simulink model "Mod4VidAincomplete"  (R2022b)
settings: Solver=FixedStepAuto  StartTime=0.0  StopTime=inf  RelTol=1e-3  EnableMultiTasking=on
libraries: vexarmcortexlib x21, RoboticsPlayground x1, vexcommonlib x1
settings Model: Creator=carol  LastModifiedBy=carol
settings DataIOCC: LimitDataPoints=on  SignalLoggingSaveFormat=ModelDataLogs  ReturnWorkspaceOutputs=off
settings OptimizationCC: ExpressionDepthLimit=2147483647  LifeSpan=Inf  MaxStackSize=64  EfficientTunableParamExpr=on
settings DebuggingCC: UnderspecifiedInitializationDetection=Classic  MergeDetectMultiDrivingBlocksExec=none  InheritedTsInSrcMsg=none  FcnCallInpInsideContextMsg=warning  StateNameClashWarn=warning  SFUnexpectedBacktrackingDiag=warning  SFNoUnconditionalDefaultTransitionDiag=warning  SFExecutionAtInitializationDiag=none  SFMachineParentedDataDiag=warning  ArithmeticOperatorsInVariantConditions=warning
settings HardwareCC: ProdBitPerPointer=32  ProdBitPerSizeT=32  ProdBitPerPtrDiffT=32  ProdLargestAtomicInteger=Long  ProdLargestAtomicFloat=Double  ProdIntDivRoundTo=Undefined  ProdWordSize=32  ProdHWDeviceType=ARM Compatible->ARM Cortex
settings ModelReferenceCC: EnableRefExpFcnMdlSchedulingChecks=on  PropagateSignalLabelsOutOfModel=off
settings SFSimCC: MATLABDynamicMemAlloc=off  CustomCodeUndefinedFunction=UseInterfaceOnly
settings RTWCC: Description=Embedded Coder  SystemTargetFile=ert.tlc  HardwareBoard=ARM Cortex-based VEX Microcontroller  TemplateMakefile=ert_default_tmf  Toolchain=GNU Tools for VEX ARM Cortex
settings CodeAppCC: IgnoreCustomStorageClasses=off  CustomSymbolStrType=$N$R$M  StateflowObjectComments=on  InternalIdentifier=Classic
settings ERTTargetCC: CodeReplacementLibrary=GCC ARM Cortex-M3  MultiwordLength=2048  ConvertIfToSwitch=off  SuppressUnreachableDefaultCases=off

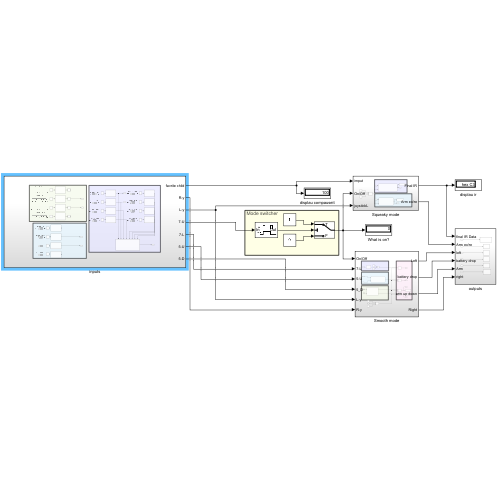
[thumbnail: Simulink's stored preview of the top-level diagram]
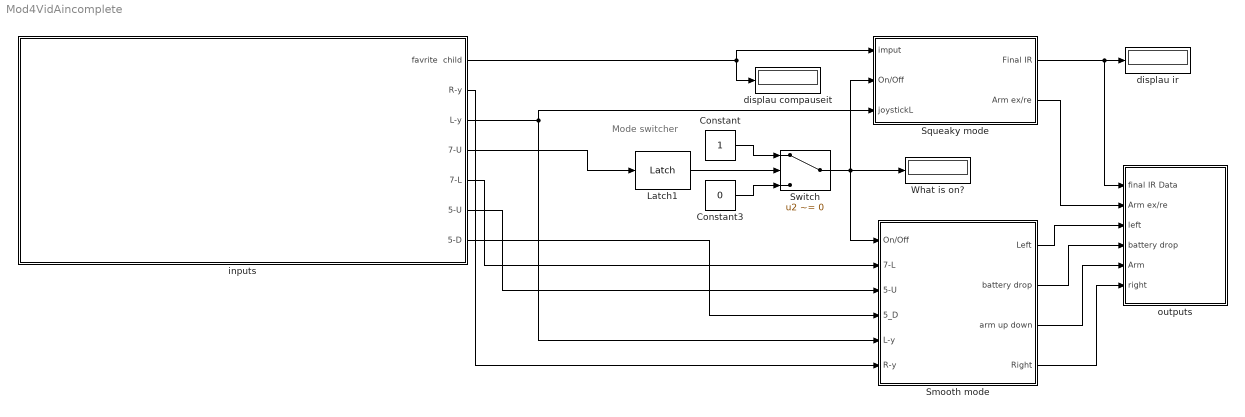
== system Mod4VidAincomplete ==
  note: Mode switcher
  Constant : Constant
  Constant3 : Constant  Value=0
  Latch1 : RoboticsPlayground/Utilities and Hardware/Latch  SystemSampleTime=-1  VariantActivationTime=update diagram  Latency=0  AutoFrameSizeCalculation=off
      settings: SourceProductName=Robotics Playground
  Smooth mode : Subsystem
  Squeaky mode : Subsystem
  Switch : Switch  Criteria=u2 ~= 0  SaturateOnIntegerOverflow=off  InputSameDT=off
  What is on? : Display
  displau compauseit : Display
  displau ir : Display
      settings: Format=hex (Stored Integer)
  inputs : Subsystem
  outputs : Subsystem
  wires:
  Switch/1 -> Squeaky mode/2(On/Off), What is on?/1, Smooth mode/1(On/Off)
  Constant3/1 -> Switch/3
  Latch1/1 -> Switch/2
  inputs/1(favrite  child) -> Squeaky mode/1(imput), displau compauseit/1
  inputs/4(7-U) -> Latch1/1
  Constant/1 -> Switch/1
  inputs/3(L-y) -> Squeaky mode/3(joystickL), Smooth mode/5(L-y)
  Smooth mode/1(Left) -> outputs/3(left)
  Smooth mode/2(battery drop) -> outputs/4(battery drop)
  Smooth mode/4(Right) -> outputs/6(right)
  Smooth mode/3(arm up down) -> outputs/5("Arm ")
  inputs/2(R-y) -> Smooth mode/6(R-y)
  inputs/7(5-D) -> Smooth mode/4(5_D)
  inputs/6(5-U) -> Smooth mode/3(5-U)
  inputs/5(7-L) -> Smooth mode/2(7-L)
  Squeaky mode/1(Final IR) -> displau ir/1, outputs/1(final IR Data)
  Squeaky mode/2(Arm ex/re) -> outputs/2(Arm ex/re)

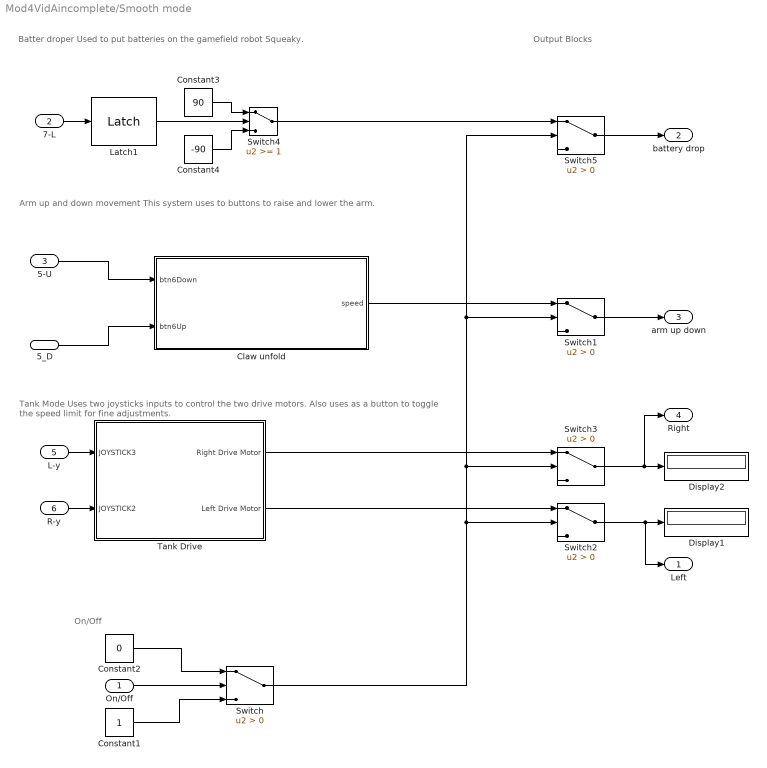
== system Mod4VidAincomplete/Smooth mode ==
  note: Output Blocks
  note: Batter droper
      | Used to put batteries on the gamefield robot Squeaky.
  note: Tank Mode
      | Uses two joysticks inputs to control the two drive motors. Also uses as a button
      | to toggle the speed limit for fine adjustments.
  note: Arm up and down movement
      | This system uses to buttons to raise and lower the arm.
  note: On/Off
  On/Off : Inport
  7-L : Inport  Port=2
  5-U : Inport  Port=3
  5_D : Inport  Port=4
  L-y : Inport  Port=5
  R-y : Inport  Port=6
  Claw unfold : Stateflow chart  TreatAsAtomicUnit=on
  Constant1 : Constant
  Constant2 : Constant  Value=0
  Constant3 : Constant  Value=90
  Constant4 : Constant  Value=-90
  Display1 : Display
  Display2 : Display
  Latch1 : vexcommonlib/Latch  output0=off  BlockPlatform=vexarmcortex
  Switch{,1..3,5} (5 alike) : Switch  Criteria=u2 > Threshold  SaturateOnIntegerOverflow=off  InputSameDT=off
  Switch4 : Switch  Threshold=1  SaturateOnIntegerOverflow=off  InputSameDT=off
  "Tank Drive " : Subsystem  TreatAsAtomicUnit=on
  Left : Outport
  battery drop : Outport  Port=2
  arm up down : Outport  Port=3
  Right : Outport  Port=4
  wires:
  Constant2/1 -> Switch/1
  On/Off/1 -> Switch/2
  5_D/1 -> Claw unfold/2(btn6Up)
  5-U/1 -> Claw unfold/1(btn6Down)
  Latch1/1 -> Switch4/2
  Constant4/1 -> Switch4/3
  R-y/1 -> "Tank Drive "/2(JOYSTICK2)
  "Tank Drive "/1(Right Drive Motor) -> Switch3/1
  L-y/1 -> "Tank Drive "/1(JOYSTICK3)
  7-L/1 -> Latch1/1
  Claw unfold/1(speed) -> Switch1/1
  Constant3/1 -> Switch4/1
  "Tank Drive "/2(Left Drive Motor) -> Switch2/1
  Switch4/1 -> Switch5/1
  Switch/1 -> Switch2/2, Switch3/2, Switch5/2, Switch1/2
  Switch5/1 -> battery drop/1
  Switch1/1 -> arm up down/1
  Switch3/1 -> Right/1, Display2/1
  Switch2/1 -> Left/1, Display1/1
  Constant1/1 -> Switch/3

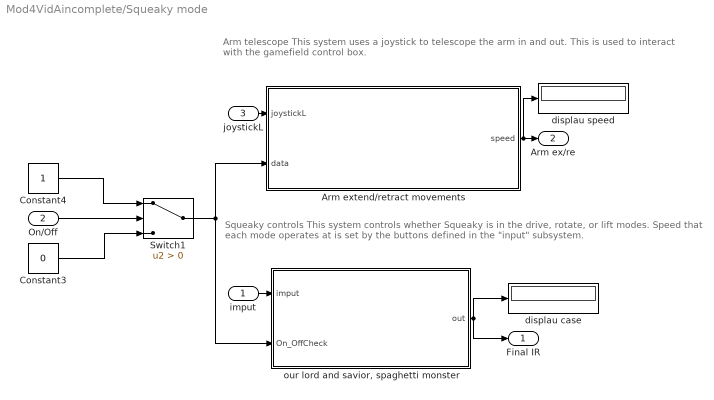
== system Mod4VidAincomplete/Squeaky mode ==
  note: Squeaky controls
      | This system controls whether Squeaky is in the drive, rotate, or lift modes.
      | Speed that each mode operates at is set by the buttons defined in the "input" subsystem.
  note: Arm telescope
      | This system uses a joystick to telescope the arm in and out.
      | This is used to interact with the gamefield control box.
  imput : Inport
  On/Off : Inport  Port=2
  joystickL : Inport  Port=3
  Arm extend/retract movements : Stateflow chart  TreatAsAtomicUnit=on
  Constant3 : Constant  Value=0
  Constant4 : Constant
  Switch1 : Switch  Criteria=u2 > Threshold  SaturateOnIntegerOverflow=off  InputSameDT=off
  displau case : Display
  displau speed : Display
  "our lord and savior, spaghetti monster" : Stateflow chart  TreatAsAtomicUnit=on
  Final IR : Outport
  Arm ex/re : Outport  Port=2
  wires:
  Switch1/1 -> Arm extend/retract movements/2(data), "our lord and savior, spaghetti monster"/2(On_OffCheck)
  imput/1 -> "our lord and savior, spaghetti monster"/1(imput)
  Constant3/1 -> Switch1/3
  joystickL/1 -> Arm extend/retract movements/1(joystickL)
  Arm extend/retract movements/1(speed) -> Arm ex/re/1, displau speed/1
  On/Off/1 -> Switch1/2
  Constant4/1 -> Switch1/1
  "our lord and savior, spaghetti monster"/1(out) -> Final IR/1, displau case/1

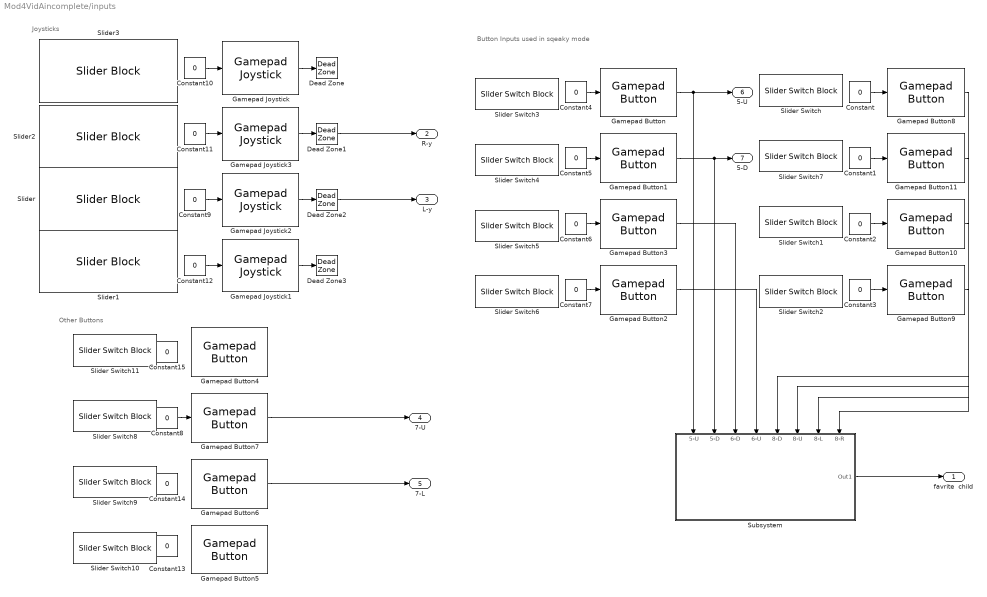
== system Mod4VidAincomplete/inputs ==
  note: Other Buttons
  note: Button Inputs used in sqeaky mode
  note: Joysticks
  Constant{,1..15} (16 alike) : Constant  Value=0
  Dead Zone{,1..3} (4 alike) : DeadZone  LowerValue=-10  UpperValue=10
  Gamepad Button : vexarmcortexlib/Gamepad/Gamepad Button  joystick=1  chan=5  button56=Up  button78=Down  SimulationIn=on  SampleTime=0.02
  Gamepad Button1 : vexarmcortexlib/Gamepad/Gamepad Button  joystick=1  chan=5  button56=Down  button78=Down  SimulationIn=on  SampleTime=0.02
  Gamepad Button10 : vexarmcortexlib/Gamepad/Gamepad Button  joystick=1  chan=8  button56=Up  button78=Left  SimulationIn=on  SampleTime=0.02
  Gamepad Button11 : vexarmcortexlib/Gamepad/Gamepad Button  joystick=1  chan=8  button56=Up  button78=Up  SimulationIn=on  SampleTime=0.02
  Gamepad Button2 : vexarmcortexlib/Gamepad/Gamepad Button  joystick=1  chan=6  button56=Up  button78=Down  SimulationIn=on  SampleTime=0.02
  Gamepad Button3 : vexarmcortexlib/Gamepad/Gamepad Button  joystick=1  chan=6  button56=Down  button78=Down  SimulationIn=on  SampleTime=0.02
  Gamepad Button4 : vexarmcortexlib/Gamepad/Gamepad Button  joystick=1  chan=7  button56=Up  button78=Down  SimulationIn=off  SampleTime=0.02
  Gamepad Button5 : vexarmcortexlib/Gamepad/Gamepad Button  joystick=1  chan=7  button56=Up  button78=Right  SimulationIn=off  SampleTime=0.02
  Gamepad Button6 : vexarmcortexlib/Gamepad/Gamepad Button  joystick=1  chan=7  button56=Up  button78=Left  SimulationIn=off  SampleTime=0.02
  Gamepad Button7 : vexarmcortexlib/Gamepad/Gamepad Button  joystick=1  chan=7  button56=Up  button78=Up  SimulationIn=on  SampleTime=0.02
  Gamepad Button8 : vexarmcortexlib/Gamepad/Gamepad Button  joystick=1  chan=8  button56=Up  button78=Down  SimulationIn=on  SampleTime=0.02
  Gamepad Button9 : vexarmcortexlib/Gamepad/Gamepad Button  joystick=1  chan=8  button56=Up  button78=Right  SimulationIn=on  SampleTime=0.02
  Gamepad Joystick : vexarmcortexlib/Gamepad/Gamepad Joystick  joystick=1  chan=1  SimulationIn=on  SampleTime=0.02
  Gamepad Joystick1 : vexarmcortexlib/Gamepad/Gamepad Joystick  joystick=1  chan=4  SimulationIn=on  SampleTime=0.02
  Gamepad Joystick2 : vexarmcortexlib/Gamepad/Gamepad Joystick  joystick=1  chan=3  SimulationIn=on  SampleTime=0.02
  Gamepad Joystick3 : vexarmcortexlib/Gamepad/Gamepad Joystick  joystick=1  chan=2  SimulationIn=on  SampleTime=0.02
  Slider{,1..3} (4 alike) : SliderBlock  ScaleMin=-180  ScaleMax=180
  Slider Switch{,1..11} (12 alike) : SliderSwitchBlock
      settings: Values={{'Off', 'On'}, [0 1]}
  Subsystem : Subsystem
      settings: PortSchema="{\"entries\":[{\"content\":{\"sides\":[{\"content\":{\"connectorIds\":[]},\"type\":\"ConnectorPlacement.EquallySpacedRectSide\",\"uuid\":\"9d2b5337-c4d4-4923-a699-a47fc21a7185\"},{\"content\":{\"connectorIds\":[\"Out1\"],\"side\":\"RIGHT\"},\"type\":\"ConnectorPlacement.EquallySpacedRectSide\",\"uuid\":\"56c06069-3940-4c56-b8fd-a4c3d4ffc63d\"},{\"content\":{\"connectorIds\":[\"In1\",\"In2\",\"In3\",\"In4\",\"In5\",\"In6\",\"In7\",\"In8\"],\"side\":\"TOP\"},\"type\":\"ConnectorPlacement.EquallySpacedRectSide\",\"uuid\":\"14368183-39e9-4405-bfbf-e8557249760c\"}]},\"type\":\"ConnectorPlacement.EquallySpacedConnector\",\"uuid\":\"5d0b0675-df6a-4749-851b-50901843da5f\"}],\"packageUris\":[\"http://schema.mathworks.com/mf0/Connector/R2020b\"],\"version\":\"1.0\"}"
  favrite  child : Outport
  R-y : Outport  Port=2
  L-y : Outport  Port=3
  7-U : Outport  Port=4
  7-L : Outport  Port=5
  5-U : Outport  Port=6
  5-D : Outport  Port=7
  wires:
  Gamepad Joystick/1 -> Dead Zone/1
  Gamepad Button7/1 -> 7-U/1
  Gamepad Button6/1 -> 7-L/1
  Constant/1 -> Gamepad Button8/1
  Constant1/1 -> Gamepad Button11/1
  Constant2/1 -> Gamepad Button10/1
  Constant3/1 -> Gamepad Button9/1
  Constant4/1 -> Gamepad Button/1
  Constant5/1 -> Gamepad Button1/1
  Constant7/1 -> Gamepad Button2/1
  Constant6/1 -> Gamepad Button3/1
  Constant8/1 -> Gamepad Button7/1
  Subsystem/1(Out1) -> favrite  child/1
  Constant9/1 -> Gamepad Joystick2/1
  Gamepad Button/1 -> 5-U/1, Subsystem/1(5-U)
  Gamepad Button1/1 -> 5-D/1, Subsystem/2(5-D)
  Gamepad Button3/1 -> Subsystem/3(6-D)
  Gamepad Button2/1 -> Subsystem/4(6-U)
  Gamepad Button8/1 -> Subsystem/5(8-D)
  Gamepad Button11/1 -> Subsystem/6(8-U)
  Gamepad Button10/1 -> Subsystem/7(8-L)
  Gamepad Button9/1 -> Subsystem/8(8-R)
  Constant12/1 -> Gamepad Joystick1/1
  Constant11/1 -> Gamepad Joystick3/1
  Constant10/1 -> Gamepad Joystick/1
  Gamepad Joystick3/1 -> Dead Zone1/1
  Gamepad Joystick2/1 -> Dead Zone2/1
  Dead Zone2/1 -> L-y/1
  Dead Zone1/1 -> R-y/1
  Gamepad Joystick1/1 -> Dead Zone3/1

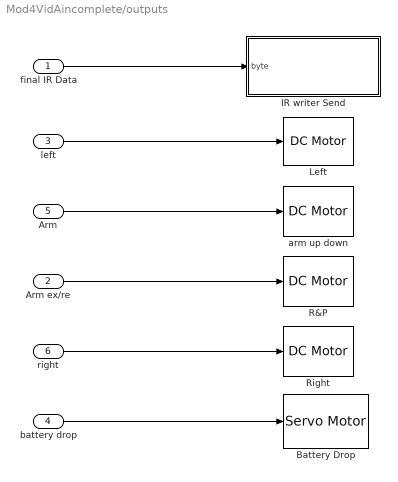
== system Mod4VidAincomplete/outputs ==
  final IR Data : Inport
  Arm ex/re : Inport  Port=2
  left : Inport  Port=3
  battery drop : Inport  Port=4
  "Arm " : Inport  Port=5
  right : Inport  Port=6
  Battery Drop : vexarmcortexlib/Actuators/Servo Motor  motor=3  scaleFactor=60/127  SimulationOut=off
  IR writer Send : Subsystem
  Left : vexarmcortexlib/Actuators/DC Motor  motor=2  scaleFactor=1/13.5  SimulationOut=off
  R&P : vexarmcortexlib/Actuators/DC Motor  motor=6  scaleFactor=1/13.5  SimulationOut=off
  Right : vexarmcortexlib/Actuators/DC Motor  motor=9  scaleFactor=1/13.5  SimulationOut=off
  arm up down : vexarmcortexlib/Actuators/DC Motor  motor=4  scaleFactor=1/13.5  SimulationOut=off
  wires:
  final IR Data/1 -> IR writer Send/1(byte)
  Arm ex/re/1 -> R&P/1
  left/1 -> Left/1
  battery drop/1 -> Battery Drop/1
  right/1 -> Right/1
  "Arm "/1 -> arm up down/1

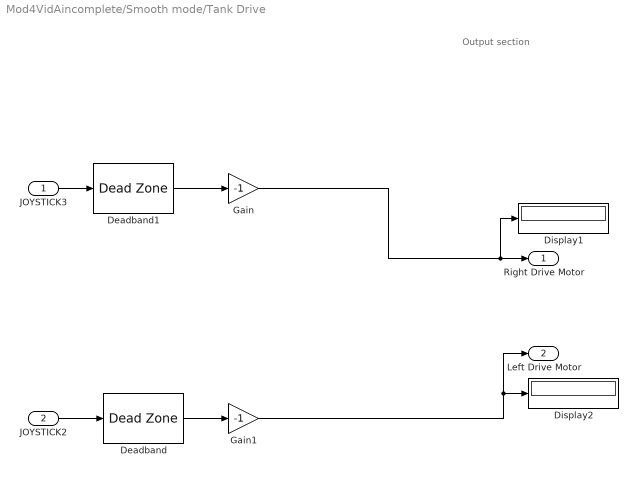
== system Mod4VidAincomplete/Smooth mode/Tank Drive  ==
  note: Output section
  JOYSTICK3 : Inport
  JOYSTICK2 : Inport  Port=2
  Deadband : DeadZone  LowerValue=-9  UpperValue=9
  Deadband1 : DeadZone  LowerValue=-9  UpperValue=9
  Display1 : Display
  Display2 : Display
  Gain : Gain  Gain=-1
  Gain1 : Gain  Gain=-1
  Right Drive Motor : Outport
  Left Drive Motor : Outport  Port=2
  wires:
  JOYSTICK3/1 -> Deadband1/1
  Gain/1 -> Display1/1, Right Drive Motor/1
  Gain1/1 -> Display2/1, Left Drive Motor/1
  JOYSTICK2/1 -> Deadband/1
  Deadband1/1 -> Gain/1
  Deadband/1 -> Gain1/1

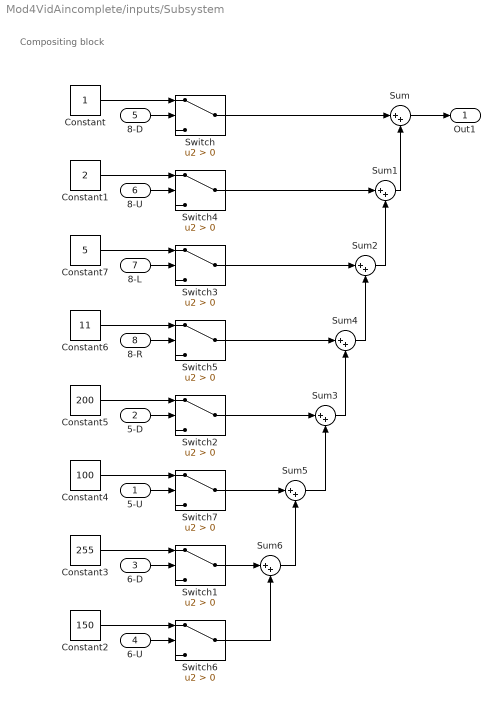
== system Mod4VidAincomplete/inputs/Subsystem ==
  note: Compositing block
  5-U : Inport
  5-D : Inport  Port=2
  6-D : Inport  Port=3
  6-U : Inport  Port=4
  8-D : Inport  Port=5
  8-U : Inport  Port=6
  8-L : Inport  Port=7
  8-R : Inport  Port=8
  Constant : Constant
  Constant1 : Constant  Value=2
  Constant2 : Constant  Value=150
  Constant3 : Constant  Value=255
  Constant4 : Constant  Value=100
  Constant5 : Constant  Value=200
  Constant6 : Constant  Value=11
  Constant7 : Constant  Value=5
  Sum{,1..6} (7 alike) : Sum  Inputs=|++
  Switch{,1..7} (8 alike) : Switch  Criteria=u2 > Threshold  SaturateOnIntegerOverflow=off  InputSameDT=off
  Out1 : Outport
  wires:
  8-D/1 -> Switch/2
  Sum/1 -> Out1/1
  Switch4/1 -> Sum1/1
  Sum1/1 -> Sum/2
  Switch3/1 -> Sum2/1
  Sum2/1 -> Sum1/2
  Switch5/1 -> Sum4/1
  Switch6/1 -> Sum6/2
  Switch1/1 -> Sum6/1
  Switch7/1 -> Sum5/1
  Switch2/1 -> Sum3/1
  Sum4/1 -> Sum2/2
  Sum3/1 -> Sum4/2
  Sum5/1 -> Sum3/2
  Sum6/1 -> Sum5/2
  Switch/1 -> Sum/1
  8-U/1 -> Switch4/2
  8-L/1 -> Switch3/2
  6-U/1 -> Switch6/2
  6-D/1 -> Switch1/2
  5-U/1 -> Switch7/2
  5-D/1 -> Switch2/2
  8-R/1 -> Switch5/2
  Constant/1 -> Switch/1
  Constant1/1 -> Switch4/1
  Constant7/1 -> Switch3/1
  Constant5/1 -> Switch2/1
  Constant6/1 -> Switch5/1
  Constant2/1 -> Switch6/1
  Constant4/1 -> Switch7/1
  Constant3/1 -> Switch1/1

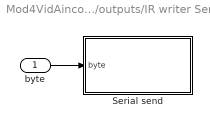
== system Mod4VidAincomplete/outputs/IR writer Send ==
  byte : Inport  OutDataTypeStr=uint8  PortDimensions=[1 1]
  Serial send : MATLAB Function  TreatAsAtomicUnit=on
  wires:
  byte/1 -> Serial send/1(byte)

== stateflow chart Mod4VidAincomplete/Smooth mode/Claw unfold ==
  state ARMDOWN
    entry:
    speed = -50;
  state STOPPED
    entry:
    speed = 0;
  state ARMUP
    entry:
    speed = 140;
  (default) -> STOPPED
  STOPPED -> ARMUP [order 1] : [btn6Down == 0 && btn6Up == 1 ]
  STOPPED -> ARMDOWN [order 2] : [btn6Down == 1 && btn6Up == 0]
  ARMDOWN -> STOPPED [order 2] : [btn6Down == 0]
  ARMUP -> STOPPED [order 2] : [btn6Up == 0]
  ARMDOWN -> STOPPED [order 1] : [btn6Down == 1 && btn6Up == 1]
  ARMUP -> STOPPED [order 1] : [btn6Down == 1 && btn6Up == 1]
  data: speed output; btn6Down input; btn6Up input

== stateflow chart Mod4VidAincomplete/Squeaky mode/Arm extend//retract movements ==
  state armExtend
    entry:
    speed = 80;
  state noArm
    entry:
    speed = 0;
  state armRetract
    entry:
    speed = -80;
  (default) -> noArm
  noArm -> armRetract [order 1] : [joystickL <= -10 && data == 1]
  noArm -> armExtend [order 2] : [joystickL >= 10 && data == 1]
  armRetract -> noArm : [joystickL == 0]
  armExtend -> noArm : [joystickL == 0]
  data: speed output; joystickL input; data input

== matlab function Mod4VidAincomplete/outputs/IR writer Send/Serial send ==
  data: byte input
function fcn(byte)
% Serial send single byte
%#codegen

% Config
port = 'uart1';
baud = uint32(9600);

persistent isFirstRun

if coder.target('Rtw')
    coder.cinclude('API.h');
    coder.cinclude('string.h');
    file = coder.opaque('FILE *', port,'HeaderFile','API.h');

    if isempty(isFirstRun)
        % first time setup
        isFirstRun = false;

        flags = coder.opaque('uint16', 'SERIAL_8N1');
        coder.ceval('usartInit', file, baud, flags);
    end

    coder.ceval('fputc', byte, file);

end

end

== stateflow chart Mod4VidAincomplete/Squeaky mode/our lord and savior, spaghetti monster ==
  state Speed Adjustments [group]
    state nyoomHigh
      entry:
      out = 0xC3;
    state nyoomLow
      entry:
      out = 0x99;
    state nyoomMed
      entry:
      out = 0xA5;
  state onOff
  state Squeaky Movements [group]
    state lift_2
      entry:
      out = 0x5A;
    state drive_2
      entry:
      out = 0x3C;
    state rotate_2
      entry:
      out = 0x33;
  state irTestDefault
    entry:
    out = 0xF0;
  state Rotational Adjustments [group]
    state spinspinHigh
      entry:
      out = 0x0F;
    state spinspinLow
      entry:
      out = 0x69;
    state spinspinMed
      entry:
      out = 0x96;
  (default) -> onOff
  irTestDefault -> nyoomHigh [order 4] : [imput == 100]
  nyoomHigh -> irTestDefault : [imput ~= 100]
  onOff -> irTestDefault : [On_OffCheck == 1]
  irTestDefault -> lift_2 [order 1] : [imput == 5]
  irTestDefault -> nyoomLow [order 7] : [imput == 200]
  lift_2 -> irTestDefault : [imput ~= 5]
  nyoomLow -> irTestDefault : [imput ~= 200]
  irTestDefault -> nyoomMed [order 8] : [imput==300]
  nyoomMed -> irTestDefault : [imput ~= 300]
  spinspinHigh -> irTestDefault : [imput ~= 150]
  irTestDefault -> drive_2 [order 2] : [imput == 1]
  drive_2 -> irTestDefault : [imput ~=1]
  irTestDefault -> spinspinHigh [order 6] : [imput == 150]
  irTestDefault -> spinspinLow [order 5] : [imput == 255]
  spinspinLow -> irTestDefault : [imput ~= 250]
  irTestDefault -> spinspinMed [order 9] : [imput == 405]
  spinspinMed -> irTestDefault : [imput ~= 405]
  rotate_2 -> irTestDefault : [imput ~= 11]
  irTestDefault -> rotate_2 [order 3] : [imput == 11]
  data: imput input; out output; On_OffCheck input
